simulink model "Adaptive Noise Cancellation"  (R2021b)
settings: Solver=FixedStepDiscrete  StartTime=0.0  StopTime=10.0  FixedStep=0.001  RelTol=1e-3
libraries: simulink x1, dspadpt3 x1
settings Model: Creator=Lenovo  LastModifiedBy=Lenovo

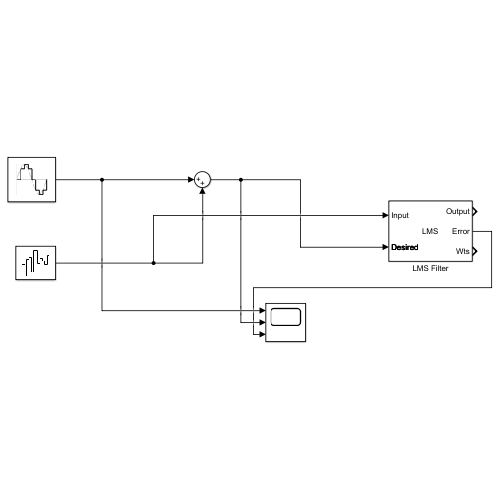
[thumbnail: Simulink's stored preview of the top-level diagram]
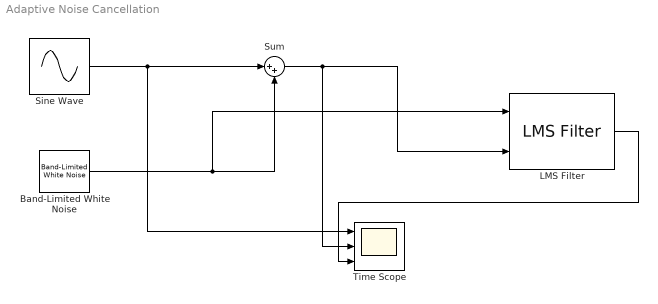
== system Adaptive Noise Cancellation ==
  Band-Limited White Noise : simulink/Sources/Band-Limited White Noise  Cov=0.001  Ts=0.001  seed=[23341]
  LMS Filter : dspadpt3/LMS Filter  Algo=LMS  L=32  stepflag=Dialog  mu=0.0001  leakage=1.0  ic=0  Adapt=off  resetflag=None  weights=on  addnparflag=off  roundingMode=Floor  overflowMode=off  secondCoeffMode=Binary point scaling  secondCoeffWordLength=2  secondCoeffFracLength=15  prodOutput2Mode=Binary point scaling  prodOutput2FracLength=20  prodOutput3Mode=Binary point scaling  prodOutput3FracLength=20  prodOutput4Mode=Binary point scaling  prodOutput4FracLength=20  quotientMode=Binary point scaling  quotientFracLength=20  accum2Mode=Binary point scaling  accum2FracLength=20
      settings: SourceProductBaseCode=DS
  Sine Wave : Sin  Frequency=2*pi*50  SampleTime=0.001
  Sum : Sum  Inputs=|++
  Time Scope : Scope  NumInputPorts=3
  wires:
  Sine Wave/1 -> Time Scope/1, Sum/1
  Band-Limited White Noise/1 -> LMS Filter/1, Sum/2
  Sum/1 -> Time Scope/2, LMS Filter/2
  LMS Filter/2 -> Time Scope/3
